simulink model "s3a"  (Simulink 2.00)
settings: Solver=ode15s  StartTime=0.0  StopTime=10  MaxStep=0.01  RelTol=1e-6  AbsTol=1e-6
values from neighbouring files (symbols this model uses):
  Iarated = 16    [M1.M]    (also in M2.M = 33.9090909091; M3A.M; M3B.M; M4.M = 3.5)
  J = 0.8    [M1.M]    (also in M2.M = 2.5; M3A.M = 0.5; M3B.M = 0.5; M4.M = 0.015)
  Laq = 0.018    [M1.M]    (also in M2.M = 0.012; M3A.M; M3B.M; M4.M = 0.01)
  Ra = 0.24    [M1.M]    (also in M2.M = 0.3; M3A.M = 0.14; M3B.M = 0.14; M4.M = 0.6)
  Rext = 2.929    [M3A.M]
  Vbrake = 0    [M3A.M]    (also in M5.M)
  Vrated = 125    [M1.M]    (also in M2.M = 220; M3A.M; M3B.M; M4.M = 120)
  wmrated = 1750*(2*pi)/60    (= 183.259571459)    [M1.M]    (also in M2.M = 156.032435128; M3A.M; M3B.M; M4.M = 293.215314335)
settings Model: MaxOrder=3  SaveTime=off  SaveOutput=off  ConsistencyChecking=off

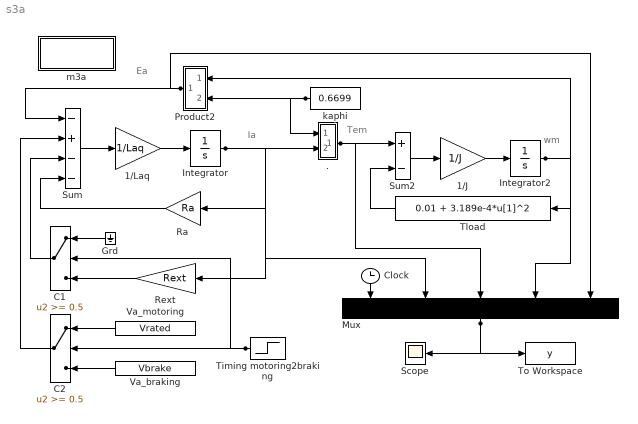
== system s3a ==
  note: Ea
  note: wm
  note: Tem
  note: Ia
  . : Subsystem
      mask Type: Dot Product
      mask Description:
      | Inner (dot) product.
      | y=sum(u1.*u2)
      mask Help: Computes the inner (dot) product of the inputs: sum(u1.*u2).  The inputs are vectors of the same length. Output is a scalar.
      mask Display: disp('.\n')
  1/J : Gain  Gain=1/J
  1/Laq : Gain  Gain=1/Laq
  C1 : Switch  Orientation=left  Threshold=0.5
  C2 : Switch  Orientation=left  Threshold=0.5
  Clock : Clock
      settings: Orientation=down  DeleteFcn=simclock BlockIsBeingDestroyed  PostSaveFcn=simclock Save
  Grd : Ground  Orientation=left
  Integrator : Integrator  ExternalReset=none  InitialConditionSource=internal  InitialCondition=Iarated  LimitOutput=off  UpperSaturationLimit=inf  LowerSaturationLimit=-inf  ShowSaturationPort=off  ShowStatePort=off  AbsoluteTolerance=auto
  Integrator2 : Integrator  ExternalReset=none  InitialConditionSource=internal  InitialCondition=wmrated  LimitOutput=off  UpperSaturationLimit=inf  LowerSaturationLimit=-inf  ShowSaturationPort=off  ShowStatePort=off  AbsoluteTolerance=auto
  m3a : Subsystem
      settings: OpenFcn=m3a
      mask Type: Masked block of m3a.m
      mask Help: Uses m3a.m to initialize and plot
      mask Display: disp('Initialize\nand plot')
  Mux : Mux  Orientation=down  Inputs=5
  Product2 : Subsystem  Orientation=left
      mask Type: Dot Product
      mask Description:
      | Inner (dot) product.
      | y=sum(u1.*u2)
      mask Help: Computes the inner (dot) product of the inputs: sum(u1.*u2).  The inputs are vectors of the same length. Output is a scalar.
      mask Display: disp('.\n')
  Ra : Gain  Orientation=left  Gain=Ra
  Rext : Gain  Orientation=left  Gain=Rext
  Scope : Scope
      settings: TickLabels=on  TimeRange=10  YMin=-300  YMax=300  SaveToWorkspace=off  SaveName=ScopeData  LimitMaxRows=off
  Sum : Sum  Inputs=-+--
  Sum2 : Sum  Inputs=+-
  Timing motoring2braking : Step  Orientation=left  Time=1  Before=1  After=0
  Tload : Fcn  Orientation=left  Expr=0.01 + 3.189e-4*u[1]^2
  To Workspace : ToWorkspace  VariableName=y  SampleTime=0
      settings: Buffer=1000
  Va_braking : Constant  Orientation=left  Value=Vbrake
  Va_motoring : Constant  Orientation=left  Value=Vrated
  kaphi : Constant  Orientation=left  Value=0.6699
  wires:
  Sum/1 -> 1/Laq/1
  Sum2/1 -> 1/J/1
  1/J/1 -> Integrator2/1
  1/Laq/1 -> Integrator/1
  Integrator/1 -> ./2(in_2), Mux/2, Ra/1, Rext/1
  Mux/1 -> To Workspace/1, Scope/1
  Clock/1 -> Mux/1
  Rext/1 -> C1/3
  kaphi/1 -> Product2/2(in_2), ./1(in_1)
  Ra/1 -> Sum/4
  C1/1 -> Sum/3
  Va_motoring/1 -> C2/1
  Va_braking/1 -> C2/3
  C2/1 -> Sum/2
  Product2/1(out_1) -> Sum/1, Mux/5
  Integrator2/1 -> Product2/1(in_1), Mux/4, Tload/1
  Timing motoring2braking/1 -> C2/2, C1/2
  ./1(out_1) -> Mux/3, Sum2/1
  Tload/1 -> Sum2/2
  Grd/1 -> C1/1

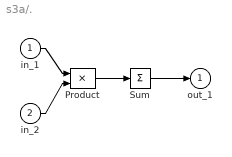
== system s3a/. ==
  in_1 : Inport  Port=1  PortWidth=-1  SampleTime=-1
  in_2 : Inport  Port=2  PortWidth=-1  SampleTime=-1
  Product : Product  Inputs=2
  Sum : Sum  Inputs=+
  out_1 : Outport  Port=1  InitialOutput=0
  wires:
  in_2/1 -> Product/2
  in_1/1 -> Product/1
  Product/1 -> Sum/1
  Sum/1 -> out_1/1

== system s3a/m3a ==
  note: Uses m3a.m to initialize and plot
      | results of S3.m

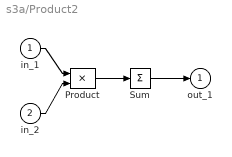
== system s3a/Product2 ==
  in_1 : Inport  Port=1  PortWidth=-1  SampleTime=-1
  in_2 : Inport  Port=2  PortWidth=-1  SampleTime=-1
  Product : Product  Inputs=2
  Sum : Sum  Inputs=+
  out_1 : Outport  Port=1  InitialOutput=0
  wires:
  in_2/1 -> Product/2
  in_1/1 -> Product/1
  Product/1 -> Sum/1
  Sum/1 -> out_1/1
